simulink model "PIcontrol_2018a"  (R2018a)
settings: Solver=VariableStepAuto  StartTime=0.0  StopTime=10.0  RelTol=1e-3
model workspace (MAT data in the model file):
  b = 50
  m = 1000
settings Model: Creator=bzhan  LastModifiedBy=bzhan
settings DataIOCC: ReturnWorkspaceOutputs=on
settings SFSimCC: SimUseLocalCustomCode=on
settings RTWCC: RTWUseLocalCustomCode=on

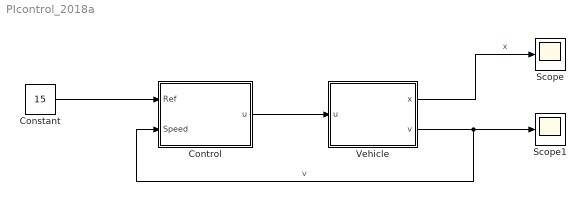
== system PIcontrol_2018a ==
  Constant : Constant  Value=15
  Control : Subsystem
  Scope : Scope
  Scope1 : Scope
  Vehicle : Subsystem
  wires:
  Constant/1 -> Control/1(Ref)
  Control/1(u) -> Vehicle/1(u)
  Vehicle/1(x) -> Scope/1  "x"
  Vehicle/2(v) -> Control/2(Speed), Scope1/1  "v"

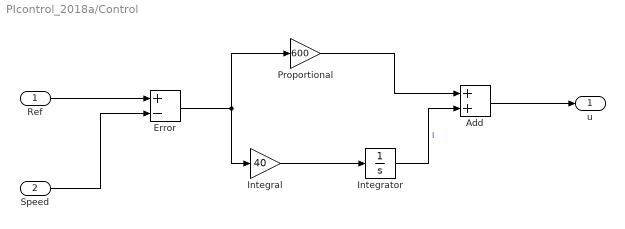
== system PIcontrol_2018a/Control ==
  Ref : Inport
  Speed : Inport  Port=2
  Add : Sum
  Error : Sum  Inputs=+-
  Integral : Gain  Gain=40
  Integrator : Integrator
  Proportional : Gain  Gain=600
  u : Outport
  wires:
  Ref/1 -> Error/1
  Speed/1 -> Error/2
  Error/1 -> Proportional/1, Integral/1
  Integral/1 -> Integrator/1
  Proportional/1 -> Add/1
  Integrator/1 -> Add/2  "I"
  Add/1 -> u/1

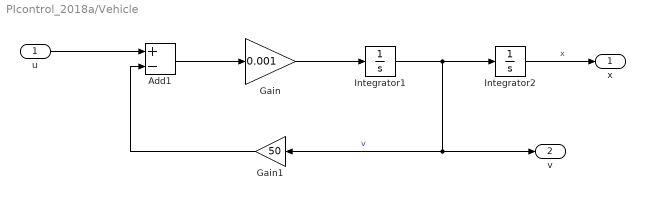
== system PIcontrol_2018a/Vehicle ==
  u : Inport
  Add1 : Sum  Inputs=+-
  Gain : Gain  Gain=0.001
  Gain1 : Gain  Gain=50
  Integrator1 : Integrator
  Integrator2 : Integrator
  x : Outport
  v : Outport  Port=2
  wires:
  u/1 -> Add1/1
  Add1/1 -> Gain/1
  Gain/1 -> Integrator1/1
  Integrator1/1 -> Gain1/1, v/1, Integrator2/1  "v"
  Integrator2/1 -> x/1  "x"
  Gain1/1 -> Add1/2
